simulink model "MissionServer_QDrone_Position_Control_FrSky"  (Simulink 9.1)
settings: Solver=ode2  StartTime=0.0  StopTime=inf  FixedStep=0.001  RelTol=1e-3  EnableMultiTasking=on
InitFcn:
  | set_param('MissionServer_QDrone_Position_Control_FrSky/MISSION SERVER QDRONE POSITION CONTROL/Trajectory Enable', 'sw', '0' )
  | set_param('MissionServer_QDrone_Position_Control_FrSky/MISSION SERVER QDRONE POSITION CONTROL/Command Enable', 'sw', '0' )
undefined symbols (not defined in the file): Host, qc_get_step_size
libraries: quarc_library x25, simulink x4
settings Model: Creator=Admin  LastModifiedBy=jpineros  SimulationMode=external  ExtModeTrigDuration=10000
settings SolverCC: PositivePriorityOrder=on
settings DataIOCC: SaveFormat=Dataset
settings OptimizationCC: LifeSpan=auto
settings DebuggingCC: UnderspecifiedInitializationDetection=Simplified  MergeDetectMultiDrivingBlocksExec=error
settings HardwareCC: ProdBitPerPointer=64  ProdBitPerSizeT=64  ProdBitPerPtrDiffT=64  ProdLargestAtomicFloat=Float  ProdIntDivRoundTo=Zero  ProdEndianess=LittleEndian  ProdWordSize=64  ProdHWDeviceType=Intel->x86-64 (Windows64)
settings ModelReferenceCC: PropagateSignalLabelsOutOfModel=on
settings RTWCC: SystemTargetFile=quarc_win64.tlc  TemplateMakefile=quarc_default_tmf  Description=QUARC Win64 Target  BuildConfiguration=Faster Runs
settings STFCustomTargetCC: ConcurrentExecutionCompliant=on  SystemTargetFile=quarc_win64.tlc
settings GRTTargetCC: TargetPreCompLibLocation=C:\PROGRA~3\QUARC\lib\2018a\win64\release  ParMdlRefBuildCompliant=off  CompOptLevelCompliant=off  MatFileLogging=off  CPPClassGenCompliant=off  UseToolchainInfoCompliant=off  ExtMode=on  ExtModeMexFile=quarc_comm
settings ConfigComp: CovHtmlReporting=off

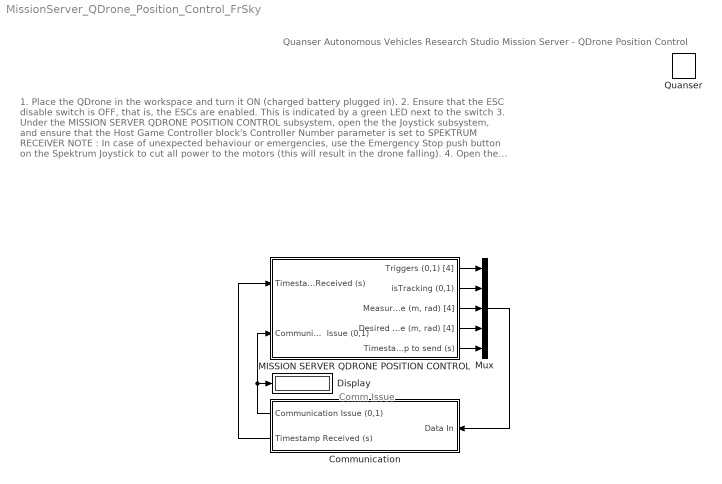
== system MissionServer_QDrone_Position_Control_FrSky ==
  note: 1. Place the QDrone in the workspace and turn it ON (charged battery plugged in).
      | 2. Ensure that the ESC disable switch is OFF, that is, the ESCs are enabled. This is indicated by a green LED next to the switch
      | 3. Under the MISSION SERVER QDRONE POSITION CONTROL subsystem, open the the Joystick subsystem, and ensure that the Host Game Controller block's Controller Number parameter is set to SPEKTRUM RECEIVER
      | NOTE : In case of unexpected behaviour or emergencies, use the Emergency Stop push button on the Spektrum Joystick to cut all power to the motors (this will result in the drone falling).
      | 4. Open the Data Server (Localization) subsystem and follow the steps there to set up the correct calibration and rigid body definition files for the selected QDrone.
      | 5. Under the QUARC menu, click on Build .
      | 6. Under the QUARC menu, click on Start . Wait for the model to start running (takes ~1 to 5 seconds for the Motive API to initialize and send localization data).
      | 7. In the MISSION SERVER QDRONE POSITION CONTROL subsystem, ensure that the isTracking? display shows 1 and that the Joystick Issue display shows 0 (joystick must be powered ON with USB dongle attached to the PC).
      | 8. Start running the Commander_Stabilizer_QDrone.mdl model.
      | 9. Arm the drone by moving the Arm/Disarm toggle to the 2 position.
      | 10. Takeoff the drone by moving the Takeoff/Land toggle to the 2 position. The QDrone should takeoff and hover.
      | 11. When finished, move the Takeoff/Land toggle to the 0 position to land the drone. The QDrone should land.
      | 12. Move the Arm/Disarm toggle to the 0 position. (The Commander_Stabilizer_QDrone.mdl model disarms the drone and stops automatically upon landing).
      | 13. Stop this model.
  note: Quanser Autonomous Vehicles Research Studio
      | Mission Server - QDrone Position Control
  note: Comm Issue
  Communication : Subsystem
  Display : Display
  MISSION SERVER QDRONE POSITION CONTROL : Subsystem
  Mux : Mux  Inputs=5
  Quanser : quarc_library/Logos/Quanser
  wires:
  Communication/2(Timestamp Received (s)) -> MISSION SERVER QDRONE POSITION CONTROL/1(Timestamp Received (s))
  MISSION SERVER QDRONE POSITION CONTROL/5(Timestamp to send (s)) -> Mux/5
  Mux/1 -> Communication/1(Data In)
  Communication/1(Communication Issue (0,1)) -> Display/1, MISSION SERVER QDRONE POSITION CONTROL/2(Communication  Issue (0,1))
  MISSION SERVER QDRONE POSITION CONTROL/3("Measured  Pose (m, rad) [4]") -> Mux/3
  MISSION SERVER QDRONE POSITION CONTROL/4("Desired  Pose (m, rad) [4]") -> Mux/4
  MISSION SERVER QDRONE POSITION CONTROL/1(Triggers (0,1) [4]) -> Mux/1
  MISSION SERVER QDRONE POSITION CONTROL/2(isTracking (0,1)) -> Mux/2

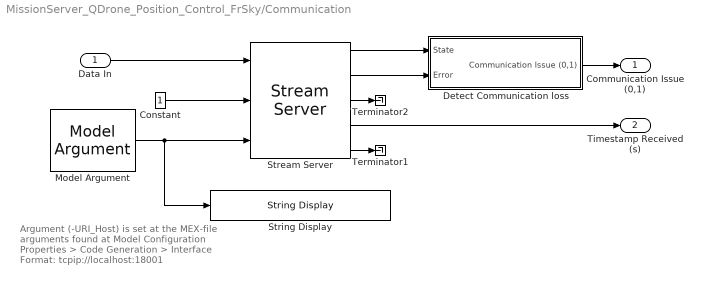
== system MissionServer_QDrone_Position_Control_FrSky/Communication ==
  note: Argument (-URI_Host) is set at the MEX-file arguments
      | found at Model Configuration Properties > Code Generation > Interface
      |
      | Format:
      | tcpip://localhost:18001
  Data In : Inport
  Constant : Constant
  Detect Communication loss : Subsystem
  Model Argument : quarc_library/Sources/Signals/Model Argument  argument_name=URI_Host  has_value=on  data_type_mode=Specify via dialog  data_type=char  max_length=80  default_value=0  variable_size=off
      settings: AttributesFormatString=(-%<argument_name>)  SourceProductName=QUARC Targets
  Stream Server : quarc_library/Communications/Basic/Stream Server  uri_source=External input port  uri=tcpip://localhost:18877  apply_uri_to_all_configs=off  send_buffer_size=1460  receive_buffer_size=1460  byte_order=little endian (Intel - LSB first)  optimization=Minimum latency  send_options=Send most recent data  receive_options=Receive most recent data  default_value=zeros(1,1)  sample_time=qc_get_step_size  active=off  implementation=Use blocking I/O in a separate thread  send_fifo_size=1000  receive_fifo_size=1000  send_priority=0  receive_priority=0  send_dimensions=off  receive_dimensions=off  max_dimensions=-1  data_type=Inherited via back propagation  type_expr=BusObject
  "String Display " : quarc_library/Strings/String Display  alignment=center  display_mode=Single line  sample_time=-1  use_new=off
      settings: SourceProductName=QUARC Targets
  Terminator1 : Terminator
  Terminator2 : Terminator
  Communication Issue (0,1) : Outport
  Timestamp Received (s) : Outport  Port=2
  wires:
  Constant/1 -> Stream Server/2
  Data In/1 -> Stream Server/1
  Stream Server/3 -> Terminator2/1
  Stream Server/5 -> Terminator1/1
  Model Argument/1 -> "String Display "/1, Stream Server/3
  Stream Server/4 -> Timestamp Received (s)/1
  Stream Server/1 -> Detect Communication loss/1(State)
  Stream Server/2 -> Detect Communication loss/2(Error)
  Detect Communication loss/1(Communication Issue (0,1)) -> Communication Issue (0,1)/1

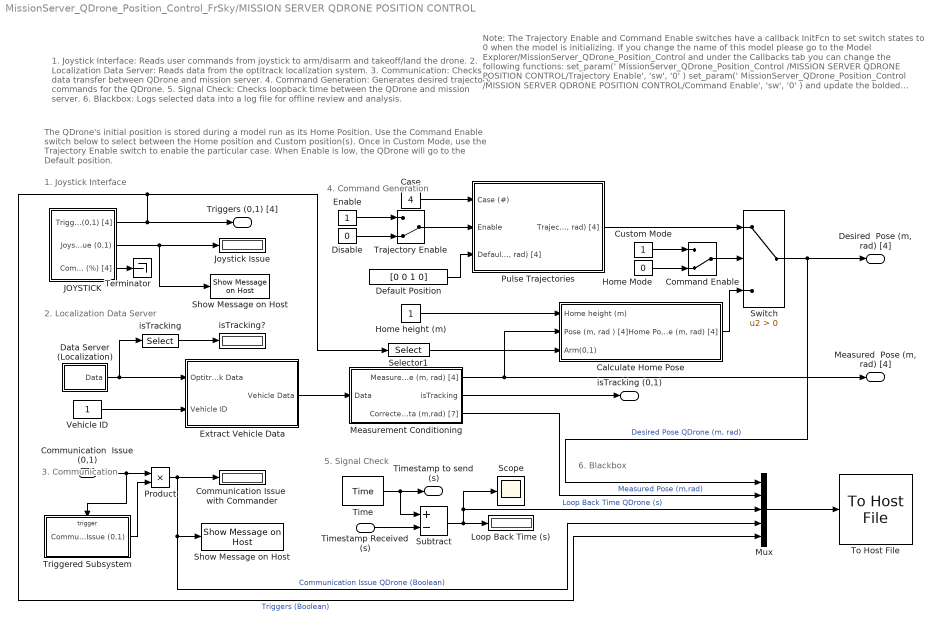
== system MissionServer_QDrone_Position_Control_FrSky/MISSION SERVER QDRONE POSITION CONTROL ==
  note: The QDrone's initial position is stored during a model run as its Home Position.
      | Use the Command Enable switch below to select between the Home position and Custom position(s).
      | Once in Custom Mode, use the Trajectory Enable switch to enable the particular case.
      | When Enable is low, the QDrone will go to the Default position.
  note: 5. Signal Check
  note: 6. Blackbox
  note: 3. Communication
  note: 2. Localization Data Server
  note: 1. Joystick Interface
  note: 4. Command Generation
  note: 1. Joystick Interface: Reads user commands from joystick to arm/disarm and takeoff/land the drone.
      | 2. Localization Data Server: Reads data from the optitrack localization system.
      | 3. Communication: Checks data transfer between QDrone and mission server.
      | 4. Command Generation: Generates desired trajectory commands for the QDrone.
      | 5. Signal Check: Checks loopback time between the QDrone and mission server.
      | 6. Blackbox: Logs selected data into a log file for offline review and analysis.
  note: Note:
      | The Trajectory Enable and Command Enable switches have a callback InitFcn to set switch states
      | to 0 when the model is initializing. If you change the name of this model please go to the Model Explorer/MissionServer_QDrone_Position_Control and under the Callbacks tab you can change the following functions:
      | set_param(' MissionServer_QDrone_Position_Control /MISSION SERVER QDRONE POSITION CONTROL/Trajectory Enable', 'sw', '0' )
      | set_param(' MissionServer_QDrone_Position_Control /MISSION SERVER QDRONE POSITION CONTROL/Command Enable', 'sw', '0' )
      | and update the bolded section with the new name of the model.
  Timestamp Received (s) : Inport
  Communication  Issue (0,1) : Inport  Port=2
  Calculate Home Pose : Subsystem
  Case : Constant  Value=4
  Command Enable : ManualSwitch  CurrentSetting=0
  Communication Issue  with Commander : Display
  Custom Mode : Constant
  "Data Server (Localization) " : Subsystem
  Default Position : Constant  Value=[0 0 1 0]
  Disable : Constant  Value=0
  Enable : Constant
  Extract Vehicle Data : Subsystem
  Home Mode : Constant  Value=0
  Home height (m) : Constant
  JOYSTICK : Subsystem
  Joystick Issue : Display
  Loop Back Time (s) : Display
  Measurement Conditioning : Subsystem
  Mux : Mux  Inputs=5
  Product : Product
  Pulse Trajectories : Subsystem
  Scope : Scope
  Selector1 : Selector  InputPortWidth=4  IndexOptions=Index vector (dialog)  Indices=[1]  OutputSizes=1
  Show Message on Host : quarc_library/Sinks/Error Handling/Show Message on Host  message_type=Fixed error message  message_icon=Warning  message=Mission Server: Communication Issue with QDrone
      settings: AttributesFormatString="\"%<message>\""  SourceProductName=QUARC Targets
  "Show Message on Host " : quarc_library/Sinks/Error Handling/Show Message on Host  message_type=Fixed error message  message_icon=Warning  message=Mission Server: Joystick Disconnected
      settings: AttributesFormatString="\"%<message>\""  SourceProductName=QUARC Targets
  Subtract : Sum  Inputs=+-
  Switch : Switch  Criteria=u2 > Threshold
  Terminator : Terminator
  Time : quarc_library/Sources/Time/Time  time_source=Wall clock  sample_time=qc_get_step_size
  To Host File : quarc_library/Sinks/To Host/To Host File  file_name=saved_data/%m/Mission_Server_%{date}_%{time}.mat  variable_name=mission_server_data  decimation=1  sample_time=-1  file_format=MAT-file v.5  options=No header or footer  append=off  final_file_name=saved_data/MissionServer_QDrone_Position_Control_FrSky/Mission_Server_20-Jan-2022_08-53-09.mat  bitrate=2000000
  Trajectory Enable : ManualSwitch  CurrentSetting=0
  Triggered Subsystem : Subsystem  TreatAsAtomicUnit=on
  Vehicle ID : Constant
  isTracking : Selector  InputPortWidth=7  IndexOptions=Index vector (dialog)  Indices=[7]  OutputSizes=1
  isTracking? : Display
  Triggers (0,1) [4] : Outport
  isTracking (0,1) : Outport  Port=2
  "Measured  Pose (m, rad) [4]" : Outport  Port=3
  "Desired  Pose (m, rad) [4]" : Outport  Port=4
  Timestamp to send (s) : Outport  Port=5
  wires:
  Communication  Issue (0,1)/1 -> Product/1, Triggered Subsystem/Trigger
  isTracking/1 -> isTracking?/1
  JOYSTICK/2(Joystick Issue (0,1)) -> "Show Message on Host "/1, Joystick Issue/1
  JOYSTICK/3(Commands (%) [4]) -> Terminator/1
  JOYSTICK/1(Triggers (0,1) [4]) -> Mux/5, Selector1/1, Triggers (0,1) [4]/1  "Triggers (Boolean)"
  Time/1 -> Subtract/1, Timestamp to send (s)/1
  Timestamp Received (s)/1 -> Subtract/2
  Subtract/1 -> Mux/3, Scope/1, Loop Back Time (s)/1  "Loop Back Time QDrone (s)"
  Switch/1 -> Mux/1, "Desired  Pose (m, rad) [4]"/1  "Desired Pose QDrone (m, rad)"
  Measurement Conditioning/2(isTracking) -> isTracking (0,1)/1
  Measurement Conditioning/1("Measured Pose (m, rad) [4]") -> Calculate Home Pose/2("Pose (m, rad ) [4]"), "Measured  Pose (m, rad) [4]"/1
  "Data Server (Localization) "/1(Data) -> Extract Vehicle Data/1(Optitrack Data), isTracking/1
  Vehicle ID/1 -> Extract Vehicle Data/2(Vehicle ID)
  Extract Vehicle Data/1(Vehicle Data) -> Measurement Conditioning/1(Data)
  Calculate Home Pose/1("Home Pose (m, rad) [4]") -> Switch/3
  Home height (m)/1 -> Calculate Home Pose/1(Home height (m))
  Triggered Subsystem/1(Communication Issue (0,1)) -> Product/2
  Product/1 -> Communication Issue  with Commander/1, Mux/4, Show Message on Host/1  "Communication Issue QDrone (Boolean)"
  Mux/1 -> To Host File/1
  Custom Mode/1 -> Command Enable/1
  Command Enable/1 -> Switch/2
  Home Mode/1 -> Command Enable/2
  Enable/1 -> Trajectory Enable/1
  Disable/1 -> Trajectory Enable/2
  Trajectory Enable/1 -> Pulse Trajectories/2(Enable)
  Default Position/1 -> Pulse Trajectories/3("Default (m, rad) [4]")
  Case/1 -> Pulse Trajectories/1(Case (#))
  Pulse Trajectories/1("Trajectory (m, rad) [4]") -> Switch/1
  Selector1/1 -> Calculate Home Pose/3(Arm(0,1))
  Measurement Conditioning/3(Corrected Pose Data (m,rad) [7]) -> Mux/2  "Measured Pose (m,rad)"

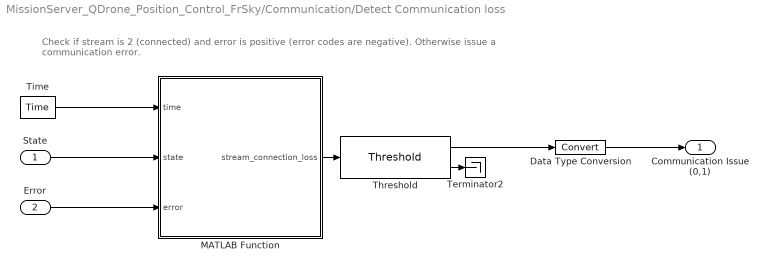
== system MissionServer_QDrone_Position_Control_FrSky/Communication/Detect Communication loss ==
  note: Check if stream is 2 (connected) and error is positive (error codes are negative). Otherwise issue a communication error.
  State : Inport
  Error : Inport  Port=2
  Data Type Conversion : DataTypeConversion
  MATLAB Function : MATLAB Function  TreatAsAtomicUnit=on
  Terminator2 : Terminator
  Threshold : quarc_library/Discontinuities/Threshold  operator=>=  param_src=Specify via dialog  threshold=0.5  duration=0.1
      settings: SourceProductName=QUARC Targets
  Time : quarc_library/Sources/Time/Time  time_source=Wall clock  sample_time=qc_get_step_size
  Communication Issue (0,1) : Outport
  wires:
  Error/1 -> MATLAB Function/3(error)
  MATLAB Function/1(stream_connection_loss) -> Threshold/1
  State/1 -> MATLAB Function/2(state)
  Time/1 -> MATLAB Function/1(time)
  Threshold/2 -> Terminator2/1
  Data Type Conversion/1 -> Communication Issue (0,1)/1
  Threshold/1 -> Data Type Conversion/1

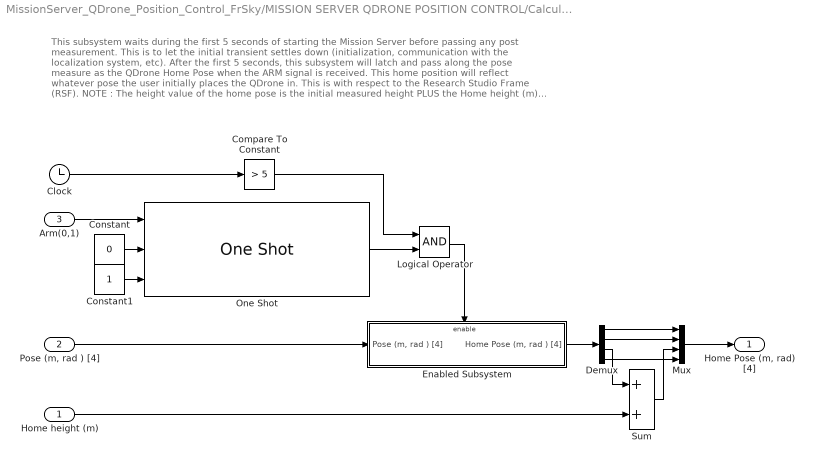
== system MissionServer_QDrone_Position_Control_FrSky/MISSION SERVER QDRONE POSITION CONTROL/Calculate Home Pose ==
  note: This subsystem waits during the first 5 seconds of starting the Mission Server before passing any post measurement.
      | This is to let the initial transient settles down (initialization, communication with the localization system, etc).
      | After the first 5 seconds, this subsystem will latch and pass along the pose measure as the QDrone Home Pose when
      | the ARM signal is received.
      | This home position will reflect whatever pose the user initially places the QDrone in.
      | This is with respect to the Research Studio Frame (RSF).
      |
      | NOTE : The height value of the home pose is the initial measured height PLUS the Home height (m) input value.
  Home height (m) : Inport
  "Pose (m, rad ) [4]" : Inport  Port=2
  Arm(0,1) : Inport  Port=3
  Clock : Clock
  Compare To Constant : simulink/Logic and Bit Operations/Compare To Constant  relop=>  const=5  OutDataTypeStr=boolean
  Constant : Constant  Value=0
  Constant1 : Constant
  Demux : Demux
  Enabled Subsystem : Subsystem  TreatAsAtomicUnit=on
  Logical Operator : Logic  AllPortsSameDT=off  OutDataTypeStr=boolean
  Mux : Mux
  One Shot : quarc_library/Discontinuities/One Shot  trigger_type=Rising edge  redun_pulse=Ignore extraneous pulse  width_source=Specify via dialog  pulse_width=1/qc_get_step_size
      settings: SourceProductName=QUARC Targets
  Sum : Sum
  "Home Pose (m, rad) [4]" : Outport
  wires:
  Constant/1 -> One Shot/2
  Constant1/1 -> One Shot/3
  Arm(0,1)/1 -> One Shot/1
  One Shot/1 -> Logical Operator/2
  "Pose (m, rad ) [4]"/1 -> Enabled Subsystem/1("Pose (m, rad ) [4] ")
  Clock/1 -> Compare To Constant/1
  Compare To Constant/1 -> Logical Operator/1
  Logical Operator/1 -> Enabled Subsystem/Enable
  Enabled Subsystem/1("Home Pose (m, rad ) [4]") -> Demux/1
  Demux/1 -> Mux/1
  Demux/2 -> Mux/2
  Demux/4 -> Mux/4
  Demux/3 -> Sum/1
  Sum/1 -> Mux/3
  Home height (m)/1 -> Sum/2
  Mux/1 -> "Home Pose (m, rad) [4]"/1

== system MissionServer_QDrone_Position_Control_FrSky/MISSION SERVER QDRONE POSITION CONTROL/Data Server (Localization)  ==
  note: Double-click on the OptiTrack Trackables block.
      |
      | Click on the ... icon under Calibration file: and select the .cal file
      | created when calibrating the Optitrack cameras
      |
      | Click on the ... icon under Trackables definition file: and select
      | the trackables file created when defining rigid bodies (for the
      | QDrone you are about to use)
  Convention Correction (Motive Frame to Research Studio Frame) : Subsystem
  Data Type Conversion : DataTypeConversion
  Mux : Mux  Inputs=3
  OptiTrack Trackables : quarc_library/Devices/Third-Party/NaturalPoint/OptiTrack/OptiTrack Trackables  calibration_file=C:\Users\user\Documents\optitrack\03-06-2020\CalibrationResult 2020-03-06 9.cal  rigid_body_file=C:\Users\user\Documents\optitrack\02-27-2020\Motive Profile - 2020-03-06.motive  rigid_body_ids=[1]  sample_time=qc_get_step_size*10  active=off
      settings: SourceProductName=QUARC Targets
  Rate Transition2 : RateTransition
  Terminator : Terminator
  Data : Outport
  wires:
  Mux/1 -> Rate Transition2/1
  Convention Correction (Motive Frame to Research Studio Frame)/1(xyz_RSF (m) [3]) -> Mux/1
  Convention Correction (Motive Frame to Research Studio Frame)/2(rot_RSF (rad) [3]) -> Mux/2
  Data Type Conversion/1 -> Mux/3
  OptiTrack Trackables/1 -> Convention Correction (Motive Frame to Research Studio Frame)/1(xyz_MF (m) [3])
  OptiTrack Trackables/2 -> Terminator/1
  OptiTrack Trackables/3 -> Convention Correction (Motive Frame to Research Studio Frame)/2(rot_MF (rad) [3])
  OptiTrack Trackables/4 -> Data Type Conversion/1
  Rate Transition2/1 -> Data/1

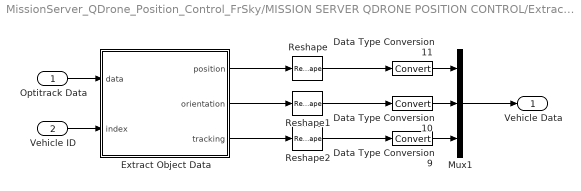
== system MissionServer_QDrone_Position_Control_FrSky/MISSION SERVER QDRONE POSITION CONTROL/Extract Vehicle Data ==
  Optitrack Data : Inport
  Vehicle ID : Inport  Port=2
  Data Type Conversion10 : DataTypeConversion
  Data Type Conversion11 : DataTypeConversion
  Data Type Conversion9 : DataTypeConversion
  Extract Object Data : MATLAB Function  TreatAsAtomicUnit=on
  Mux1 : Mux  Inputs=3
  Reshape : Reshape
  Reshape1 : Reshape
  Reshape2 : Reshape
  Vehicle Data : Outport
  wires:
  Vehicle ID/1 -> Extract Object Data/2(index)
  Optitrack Data/1 -> Extract Object Data/1(data)
  Mux1/1 -> Vehicle Data/1
  Extract Object Data/1(position) -> Reshape/1
  Extract Object Data/3(tracking) -> Reshape2/1
  Extract Object Data/2(orientation) -> Reshape1/1
  Data Type Conversion11/1 -> Mux1/1
  Data Type Conversion10/1 -> Mux1/2
  Data Type Conversion9/1 -> Mux1/3
  Reshape/1 -> Data Type Conversion11/1
  Reshape1/1 -> Data Type Conversion10/1
  Reshape2/1 -> Data Type Conversion9/1

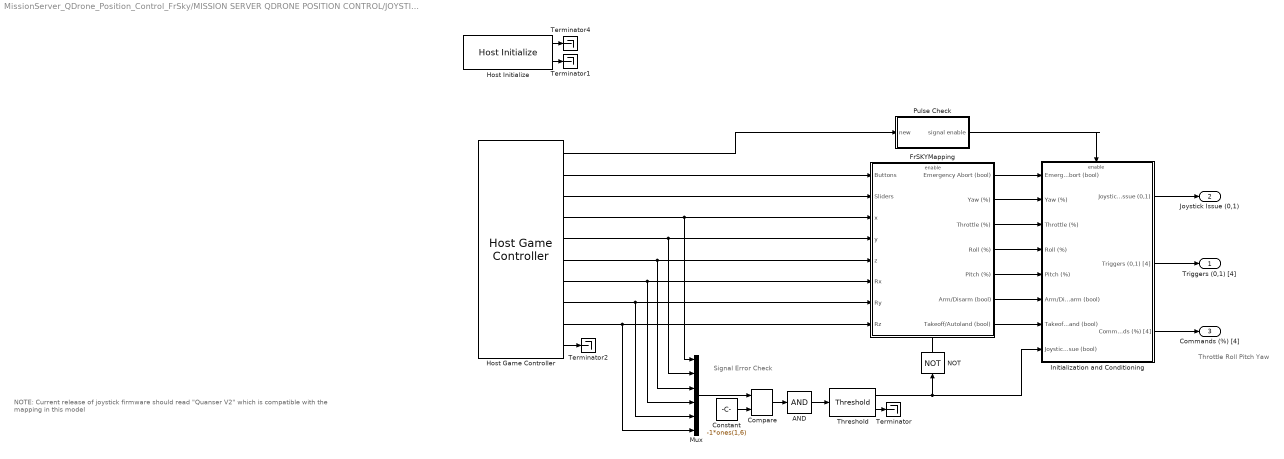
== system MissionServer_QDrone_Position_Control_FrSky/MISSION SERVER QDRONE POSITION CONTROL/JOYSTICK ==
  note: Signal Error Check
  note: Throttle
      | Roll
      | Pitch
      | Yaw
  note: NOTE: Current release of joystick firmware should read "Quanser V2" which is compatible with the mapping in this model
  AND : Logic  Inputs=1  AllPortsSameDT=off  OutDataTypeStr=boolean
  Compare : quarc_library/Logic Operations/Compare  operator===  output_data_type=boolean
      settings: SourceProductName=QUARC Targets
  Constant : Constant  Value=-1*ones(1,6)
  FrSKYMapping : Subsystem
  Host Game Controller : quarc_library/Devices/Peripherals/Host/Host Game Controller  object_name=Host-1  controller=1  buffer_size=20  deadzone=[]  saturation=[]  sample_time=qc_get_step_size  auto_center=off  enabled=on  debug_mode=off
      settings: SourceProductName=QUARC Targets
  Host Initialize : quarc_library/Devices/Peripherals/Host/Host Initialize  object_name=Host-1  uri_source=Use external mode communications  uri=tcpip://localhost:18001  apply_uri_to_all_configs=on  send_buffer_size=1000  receive_buffer_size=1000  thread_priority=0  run_client=on  use_window=off  window_position=[]  sample_time=qc_get_step_size  active=on
      settings: SourceProductName=QUARC Targets
  Initialization and Conditioning : Subsystem  TreatAsAtomicUnit=on
  Mux : Mux  Inputs=6
  NOT : Logic  Operator=NOT  IconShape=distinctive  AllPortsSameDT=off  OutDataTypeStr=boolean
  Pulse Check : Subsystem  TreatAsAtomicUnit=on
  Terminator{,1..2,4} (4 alike) : Terminator
  Threshold : quarc_library/Discontinuities/Threshold  operator=>=  param_src=Specify via dialog  threshold=0.5  duration=0.2
      settings: SourceProductName=QUARC Targets
  Triggers (0,1) [4] : Outport
  Joystick Issue (0,1) : Outport  Port=2
  Commands (%) [4] : Outport  Port=3
  wires:
  FrSKYMapping/2(Yaw (%)) -> Initialization and Conditioning/2(Yaw (%))
  FrSKYMapping/3(Throttle (%)) -> Initialization and Conditioning/3(Throttle (%))
  FrSKYMapping/1(Emergency Abort (bool)) -> Initialization and Conditioning/1(Emergency Abort (bool))
  FrSKYMapping/5(Pitch (%)) -> Initialization and Conditioning/5(Pitch (%))
  FrSKYMapping/6("Arm/Disarm (bool) ") -> Initialization and Conditioning/6(Arm/Disarm (bool))
  FrSKYMapping/4(Roll (%)) -> Initialization and Conditioning/4(Roll (%))
  Host Game Controller/1 -> Pulse Check/1(new)
  Pulse Check/1(signal enable) -> Initialization and Conditioning/Enable
  FrSKYMapping/7(Takeoff/Autoland (bool)) -> Initialization and Conditioning/7(Takeoff/AutoLand (bool))
  Host Game Controller/4 -> Mux/1, FrSKYMapping/3(x)
  Host Game Controller/5 -> Mux/2, FrSKYMapping/4(y)
  Host Game Controller/6 -> Mux/3, FrSKYMapping/5(z)
  Host Game Controller/7 -> Mux/4, FrSKYMapping/6(Rx)
  Host Game Controller/8 -> Mux/5, FrSKYMapping/7(Ry)
  Host Game Controller/9 -> Mux/6, FrSKYMapping/8(Rz)
  Mux/1 -> Compare/1
  Constant/1 -> Compare/2
  Compare/1 -> AND/1
  Threshold/2 -> Terminator/1
  Host Game Controller/2 -> FrSKYMapping/1(Buttons)
  Host Game Controller/3 -> FrSKYMapping/2(Sliders)
  Threshold/1 -> NOT/1, Initialization and Conditioning/8(Joystick Issue (bool))
  NOT/1 -> FrSKYMapping/Enable
  AND/1 -> Threshold/1
  Initialization and Conditioning/3(Commands (%) [4]) -> Commands (%) [4]/1
  Initialization and Conditioning/2(Triggers (0,1) [4]) -> Triggers (0,1) [4]/1
  Host Initialize/2 -> Terminator1/1
  Host Initialize/1 -> Terminator4/1
  Host Game Controller/10 -> Terminator2/1
  Initialization and Conditioning/1(Joystick Issue (0,1)) -> Joystick Issue (0,1)/1

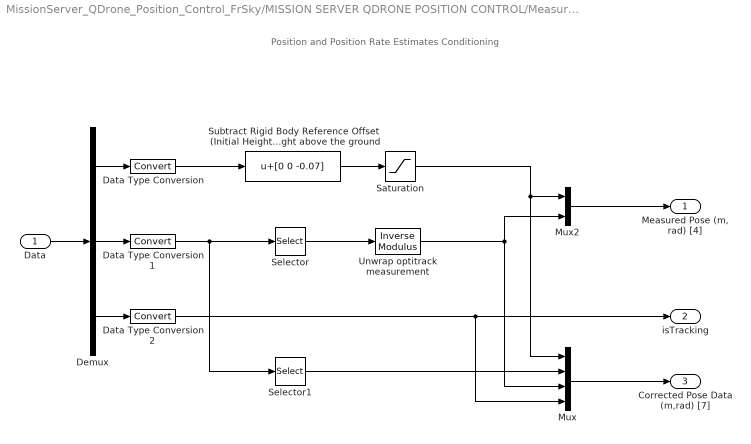
== system MissionServer_QDrone_Position_Control_FrSky/MISSION SERVER QDRONE POSITION CONTROL/Measurement Conditioning ==
  note: Position and Position Rate Estimates Conditioning
  Data : Inport
  Data Type Conversion : DataTypeConversion
  Data Type Conversion1 : DataTypeConversion
  Data Type Conversion2 : DataTypeConversion
  Demux : Demux  Outputs=[3 3 1]
  Mux : Mux
  Mux2 : Mux  Inputs=[3 1]
  Saturation : Saturate  UpperLimit=[2 2 5]  LowerLimit=[-2 -2 0]
  Selector : Selector  InputPortWidth=3  IndexOptions=Index vector (dialog)  Indices=[3]  OutputSizes=1
  Selector1 : Selector  InputPortWidth=3  IndexOptions=Index vector (dialog)  Indices=[1 2]  OutputSizes=1
  Subtract Rigid Body Reference Offset  (Initial Height)  to get height above the ground : Bias  Bias=[0 0 -0.07]
  Unwrap optitrack measurement : quarc_library/Discontinuities/Inverse Modulus  modulus=2*pi  output_derivative=off  output_revolutions=off  max_x=Inf  min_x=-Inf
  "Measured Pose (m, rad) [4]" : Outport
  isTracking : Outport  Port=2
  Corrected Pose Data (m,rad) [7] : Outport  Port=3
  wires:
  Demux/2 -> Data Type Conversion1/1
  Demux/1 -> Data Type Conversion/1
  Demux/3 -> Data Type Conversion2/1
  Mux2/1 -> "Measured Pose (m, rad) [4]"/1
  Data/1 -> Demux/1
  Data Type Conversion2/1 -> Mux/4, isTracking/1
  Subtract Rigid Body Reference Offset  (Initial Height)  to get height above the ground/1 -> Saturation/1
  Saturation/1 -> Mux2/1, Mux/1
  Data Type Conversion1/1 -> Selector1/1, Selector/1
  Selector/1 -> Unwrap optitrack measurement/1
  Data Type Conversion/1 -> Subtract Rigid Body Reference Offset  (Initial Height)  to get height above the ground/1
  Unwrap optitrack measurement/1 -> Mux/3, Mux2/2
  Mux/1 -> Corrected Pose Data (m,rad) [7]/1
  Selector1/1 -> Mux/2

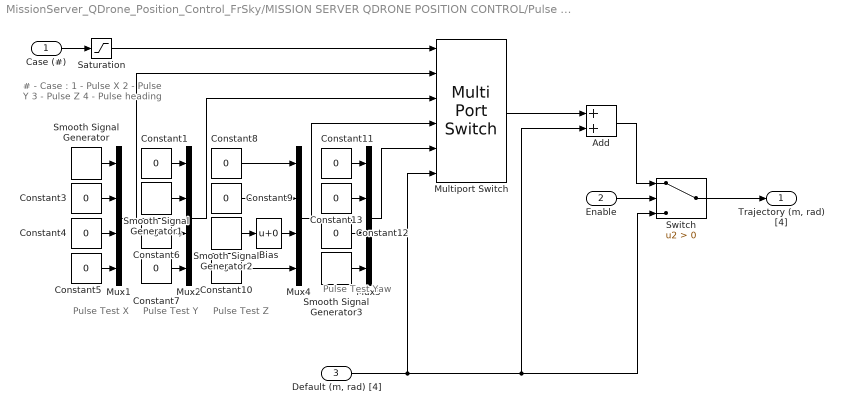
== system MissionServer_QDrone_Position_Control_FrSky/MISSION SERVER QDRONE POSITION CONTROL/Pulse Trajectories ==
  note: Pulse
      | Test Y
  note: Pulse
      | Test X
  note: Pulse
      | Test Z
  note: Pulse
      | Test
      | Yaw
  note: # - Case :
      | 1 - Pulse X
      | 2 - Pulse Y
      | 3 - Pulse Z
      | 4 - Pulse heading
  Case (#) : Inport
  Enable : Inport  Port=2
  "Default (m, rad) [4]" : Inport  Port=3
  Add : Sum
  Bias : Bias
  Constant{1,3..13} (12 alike) : Constant  Value=0
  Multiport Switch : MultiPortSwitch  Inputs=5
  Mux{1..2,4..5} (4 alike) : Mux  Inputs=[1 1 1 1]
  Saturation : Saturate  UpperLimit=5  LowerLimit=1
  Smooth Signal Generator : quarc_library/Sources/Signals/Smooth Signal Generator  signal_type=Square  source=Internal (dialog parameters)  amplitude=0.75  frequency=0.05  initial_phase=0  sample_time=qc_get_step_size  output_cos=off
      settings: SourceProductName=QUARC Targets
  Smooth Signal Generator1 : quarc_library/Sources/Signals/Smooth Signal Generator  signal_type=Square  source=Internal (dialog parameters)  amplitude=0.75  frequency=0.05  initial_phase=0  sample_time=qc_get_step_size  output_cos=off
      settings: SourceProductName=QUARC Targets
  Smooth Signal Generator2 : quarc_library/Sources/Signals/Smooth Signal Generator  signal_type=Square  source=Internal (dialog parameters)  amplitude=0.5  frequency=0.05  initial_phase=0  sample_time=qc_get_step_size  output_cos=off
      settings: SourceProductName=QUARC Targets
  Smooth Signal Generator3 : quarc_library/Sources/Signals/Smooth Signal Generator  signal_type=Square  source=Internal (dialog parameters)  amplitude=pi/4  frequency=0.05  initial_phase=0  sample_time=qc_get_step_size  output_cos=off
      settings: SourceProductName=QUARC Targets
  Switch : Switch  Criteria=u2 > Threshold
  "Trajectory (m, rad) [4]" : Outport
  wires:
  Constant3/1 -> Mux1/2
  Smooth Signal Generator/1 -> Mux1/1
  Constant5/1 -> Mux1/4
  Constant4/1 -> Mux1/3
  Mux1/1 -> Multiport Switch/2
  Case (#)/1 -> Saturation/1
  Mux2/1 -> Multiport Switch/3
  Constant6/1 -> Mux2/3
  Constant7/1 -> Mux2/4
  Constant1/1 -> Mux2/1
  Smooth Signal Generator1/1 -> Mux2/2
  Constant9/1 -> Mux4/2
  Constant8/1 -> Mux4/1
  Constant10/1 -> Mux4/4
  Smooth Signal Generator2/1 -> Bias/1
  Bias/1 -> Mux4/3
  Constant13/1 -> Mux5/2
  Constant11/1 -> Mux5/1
  Smooth Signal Generator3/1 -> Mux5/4
  Constant12/1 -> Mux5/3
  Mux4/1 -> Multiport Switch/4
  Mux5/1 -> Multiport Switch/5
  Saturation/1 -> Multiport Switch/1
  "Default (m, rad) [4]"/1 -> Add/2, Switch/3, Multiport Switch/6
  Switch/1 -> "Trajectory (m, rad) [4]"/1
  Enable/1 -> Switch/2
  Multiport Switch/1 -> Add/1
  Add/1 -> Switch/1

== system MissionServer_QDrone_Position_Control_FrSky/MISSION SERVER QDRONE POSITION CONTROL/Triggered Subsystem ==
  note: This looks for the first falling edge of the communication issue before allowing a communication issue to be triggered,
      | because the mission server model starts first.
  Trigger : TriggerPort  TriggerType=falling  VariantControl=Variant
  Add : Sum
  Compare To Constant : simulink/Logic and Bit Operations/Compare To Constant  relop=>=  const=1  OutDataTypeStr=boolean
  Constant : Constant
  Memory : Memory  InheritSampleTime=on
  Communication Issue (0,1) : Outport  InitialOutput=0
  wires:
  Constant/1 -> Add/1
  Memory/1 -> Add/2
  Add/1 -> Compare To Constant/1, Memory/1
  Compare To Constant/1 -> Communication Issue (0,1)/1

== system MissionServer_QDrone_Position_Control_FrSky/MISSION SERVER QDRONE POSITION CONTROL/Calculate Home Pose/Enabled Subsystem ==
  "Pose (m, rad ) [4] " : Inport
  Enable : EnablePort
  "Home Pose (m, rad ) [4]" : Outport
  wires:
  "Pose (m, rad ) [4] "/1 -> "Home Pose (m, rad ) [4]"/1

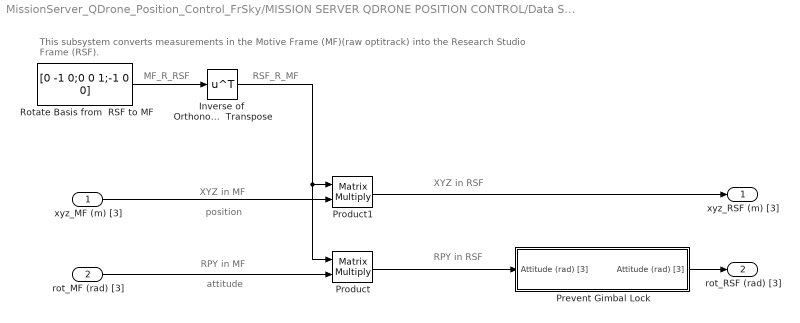
== system MissionServer_QDrone_Position_Control_FrSky/MISSION SERVER QDRONE POSITION CONTROL/Data Server (Localization) /Convention Correction (Motive Frame to Research Studio Frame) ==
  note: MF_R_RSF
  note: This subsystem converts measurements in the Motive Frame (MF)(raw optitrack) into the Research Studio Frame (RSF).
  note: RSF_R_MF
  note: XYZ in MF
  note: RPY in MF
  note: position
  note: attitude
  note: XYZ in RSF
  note: RPY in RSF
  xyz_MF (m) [3] : Inport
  rot_MF (rad) [3] : Inport  Port=2
  Inverse of  Orthonormal  Matrix is its  Transpose : Math  Operator=transpose  SaturateOnIntegerOverflow=on
  Prevent Gimbal Lock : Subsystem
  Product : Product  Multiplication=Matrix(*)
  Product1 : Product  Multiplication=Matrix(*)
  Rotate Basis from  RSF to MF : Constant  Value=[0 -1 0;0 0 1;-1 0 0]
  xyz_RSF (m) [3] : Outport
  rot_RSF (rad) [3] : Outport  Port=2
  wires:
  Rotate Basis from  RSF to MF/1 -> Inverse of  Orthonormal  Matrix is its  Transpose/1
  xyz_MF (m) [3]/1 -> Product1/2
  Inverse of  Orthonormal  Matrix is its  Transpose/1 -> Product1/1, Product/1
  rot_MF (rad) [3]/1 -> Product/2
  Product1/1 -> xyz_RSF (m) [3]/1
  Product/1 -> Prevent Gimbal Lock/1(Attitude (rad) [3])
  Prevent Gimbal Lock/1("Attitude (rad) [3] ") -> rot_RSF (rad) [3]/1

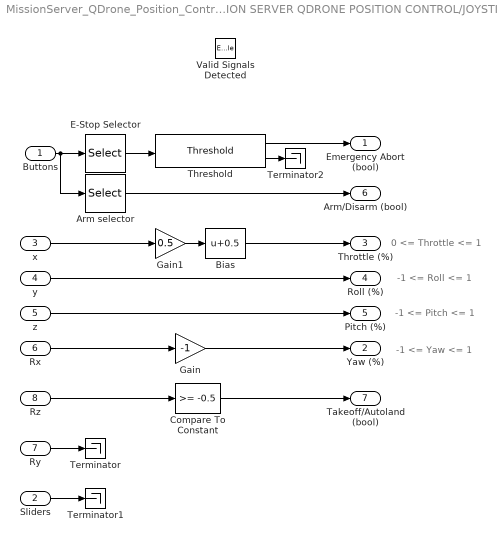
== system MissionServer_QDrone_Position_Control_FrSky/MISSION SERVER QDRONE POSITION CONTROL/JOYSTICK/FrSKYMapping ==
  note: -1 <= Yaw <= 1
  note: 0 <= Throttle <= 1
  note: -1 <= Roll <= 1
  note: -1 <= Pitch <= 1
  Buttons : Inport
  Sliders : Inport  Port=2
  x : Inport  Port=3
  y : Inport  Port=4
  z : Inport  Port=5
  Rx : Inport  Port=6
  Ry : Inport  Port=7
  Rz : Inport  Port=8
  Valid Signals Detected : EnablePort
  Arm selector : Selector  InputPortWidth=32  IndexOptions=Index vector (dialog)  Indices=[2]  OutputSizes=1
  Bias : Bias  Bias=0.5
  Compare To Constant : simulink/Logic and Bit Operations/Compare To Constant  relop=>=  const=-0.5  OutDataTypeStr=boolean
  E-Stop Selector : Selector  InputPortWidth=32  IndexOptions=Index vector (dialog)  Indices=[1]  OutputSizes=1
  Gain : Gain  Gain=-1
  Gain1 : Gain  Gain=0.5
  Terminator : Terminator
  Terminator1 : Terminator
  Terminator2 : Terminator
  Threshold : quarc_library/Discontinuities/Threshold  operator=>=  param_src=Specify via dialog  threshold=0.5  duration=0.2
      settings: SourceProductName=QUARC Targets
  Emergency Abort (bool) : Outport
  Yaw (%) : Outport  Port=2
  Throttle (%) : Outport  Port=3
  Roll (%) : Outport  Port=4
  Pitch (%) : Outport  Port=5
  "Arm/Disarm (bool) " : Outport  Port=6
  Takeoff/Autoland (bool) : Outport  Port=7
  wires:
  Buttons/1 -> Arm selector/1, E-Stop Selector/1
  Arm selector/1 -> "Arm/Disarm (bool) "/1
  x/1 -> Gain1/1
  y/1 -> Roll (%)/1
  z/1 -> Pitch (%)/1
  Rx/1 -> Gain/1
  Ry/1 -> Terminator/1
  Sliders/1 -> Terminator1/1
  E-Stop Selector/1 -> Threshold/1
  Rz/1 -> Compare To Constant/1
  Compare To Constant/1 -> Takeoff/Autoland (bool)/1
  Threshold/1 -> Emergency Abort (bool)/1
  Threshold/2 -> Terminator2/1
  Gain/1 -> Yaw (%)/1
  Gain1/1 -> Bias/1
  Bias/1 -> Throttle (%)/1

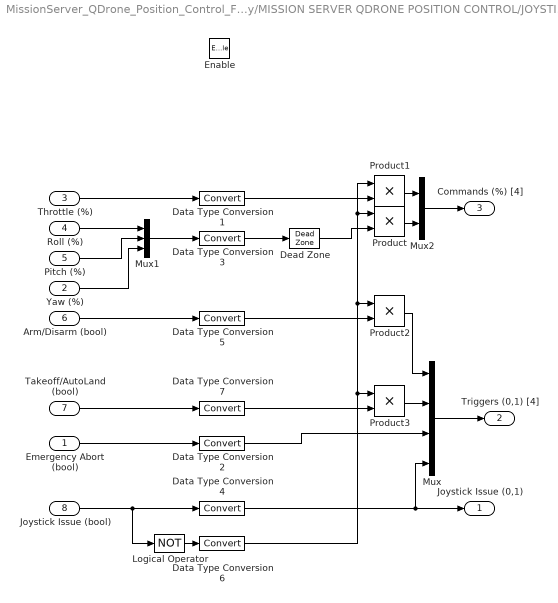
== system MissionServer_QDrone_Position_Control_FrSky/MISSION SERVER QDRONE POSITION CONTROL/JOYSTICK/Initialization and Conditioning ==
  Emergency Abort (bool) : Inport
  Yaw (%) : Inport  Port=2
  Throttle (%) : Inport  Port=3
  Roll (%) : Inport  Port=4
  Pitch (%) : Inport  Port=5
  Arm/Disarm (bool) : Inport  Port=6
  Takeoff/AutoLand (bool) : Inport  Port=7
  Joystick Issue (bool) : Inport  Port=8
  Enable : EnablePort  StatesWhenEnabling=reset
  Data Type Conversion{1..7} (7 alike) : DataTypeConversion
  Dead Zone : DeadZone  LowerValue=-0.01  UpperValue=0.01  SaturateOnIntegerOverflow=on
  Logical Operator : Logic  Operator=NOT  AllPortsSameDT=off  OutDataTypeStr=boolean
  Mux : Mux
  Mux1 : Mux  Inputs=3
  Mux2 : Mux  Inputs=2
  Product{,1..3} (4 alike) : Product
  Joystick Issue (0,1) : Outport  InitialOutput=0
  Triggers (0,1) [4] : Outport  Port=2  InitialOutput=0
  Commands (%) [4] : Outport  Port=3  InitialOutput=0
  wires:
  Joystick Issue (bool)/1 -> Data Type Conversion4/1, Logical Operator/1
  Mux1/1 -> Data Type Conversion3/1
  Throttle (%)/1 -> Data Type Conversion1/1
  Roll (%)/1 -> Mux1/1
  Pitch (%)/1 -> Mux1/2
  Yaw (%)/1 -> Mux1/3
  Data Type Conversion4/1 -> Mux/4, Joystick Issue (0,1)/1
  Emergency Abort (bool)/1 -> Data Type Conversion2/1
  Data Type Conversion3/1 -> Dead Zone/1
  Arm/Disarm (bool)/1 -> Data Type Conversion5/1
  Mux/1 -> Triggers (0,1) [4]/1
  Data Type Conversion2/1 -> Mux/3
  Logical Operator/1 -> Data Type Conversion6/1
  Product/1 -> Mux2/2
  Product1/1 -> Mux2/1
  Data Type Conversion1/1 -> Product1/2
  Dead Zone/1 -> Product/2
  Data Type Conversion6/1 -> Product1/1, Product/1, Product2/1, Product3/1
  Product2/1 -> Mux/1
  Data Type Conversion5/1 -> Product2/2
  Takeoff/AutoLand (bool)/1 -> Data Type Conversion7/1
  Product3/1 -> Mux/2
  Data Type Conversion7/1 -> Product3/2
  Mux2/1 -> Commands (%) [4]/1

== system MissionServer_QDrone_Position_Control_FrSky/MISSION SERVER QDRONE POSITION CONTROL/JOYSTICK/Pulse Check ==
  note: For this subsystem we will count the number of new pulses. The data can be considered enabled once the count of new signals has gone beyond 1. This will enable the Initializing and conditioning subsystem.
  new : Inport
  Compare : quarc_library/Logic Operations/Compare  operator=>=  output_data_type=boolean
      settings: SourceProductName=QUARC Targets
  Pulse Check : Constant
  "pulse count " : Subsystem  TreatAsAtomicUnit=on
  signal enable : Outport  InitialOutput=0
  wires:
  Compare/1 -> signal enable/1
  Pulse Check/1 -> Compare/2
  new/1 -> "pulse count "/Trigger
  "pulse count "/1(Number of Pulses) -> Compare/1

== system MissionServer_QDrone_Position_Control_FrSky/MISSION SERVER QDRONE POSITION CONTROL/Data Server (Localization) /Convention Correction (Motive Frame to Research Studio Frame)/Prevent Gimbal Lock ==
  note: Remapping the rotation order to prevent gimbal lock
      | in heading/yaw due to Euler singularity condition
  Attitude (rad) [3] : Inport
  Demux : Demux  Outputs=3
  Euler Angles from Rotation Matrix (Relative ZYX) : quarc_library/Math Operations/Matrices/Euler Angles from Rotation Matrix  menu_order=Relative Z-Y-X
      settings: SourceProductName=QUARC Targets
  Euler Angles to Rotation Matrix (Relative YZX) : quarc_library/Math Operations/Matrices/Euler Angles to Rotation Matrix  menu_order=Relative Y-Z-X
      settings: SourceProductName=QUARC Targets
  Mux : Mux  Inputs=3
  "Attitude (rad) [3] " : Outport
  wires:
  Euler Angles from Rotation Matrix (Relative ZYX)/2 -> Mux/2
  Euler Angles from Rotation Matrix (Relative ZYX)/1 -> Mux/3
  Euler Angles from Rotation Matrix (Relative ZYX)/3 -> Mux/1
  Euler Angles to Rotation Matrix (Relative YZX)/1 -> Euler Angles from Rotation Matrix (Relative ZYX)/1
  Attitude (rad) [3]/1 -> Demux/1
  Mux/1 -> "Attitude (rad) [3] "/1
  Demux/2 -> Euler Angles to Rotation Matrix (Relative YZX)/1
  Demux/3 -> Euler Angles to Rotation Matrix (Relative YZX)/2
  Demux/1 -> Euler Angles to Rotation Matrix (Relative YZX)/3

== system MissionServer_QDrone_Position_Control_FrSky/MISSION SERVER QDRONE POSITION CONTROL/JOYSTICK/Pulse Check/pulse count  ==
  Trigger : TriggerPort  TriggerType=either  VariantControl=Variant
  Constant1 : Constant  Value=0
  Increment Stored Integer : simulink/Additional Math & Discrete/Additional Math: Increment - Decrement/Increment Stored Integer
  Sum : Sum  Inputs=|++
  Unit Delay : UnitDelay  SampleTime=-1
  Number of Pulses : Outport
  wires:
  Constant1/1 -> Sum/1
  Sum/1 -> Increment Stored Integer/1
  Unit Delay/1 -> Sum/2
  Increment Stored Integer/1 -> Unit Delay/1, Number of Pulses/1

== matlab function MISSION SERVER QDRONE POSITION CONTROL/Extract Vehicle Data/Extract Object Data ==
  data: data input double; position output double; orientation output double; index input double; tracking output double
function [position, orientation, tracking] = fcn(data, index)

n = length(data)/7;

if (index<=0)||(index>n)
    position = zeros(1,3); orientation = zeros(1,3); tracking = 0;
else
    position = [data(index*3-2), data(index*3-1), data(index*3)];
    orientation = [data((index+n)*3 - 2), data((index+n)*3 - 1), data((index+n)*3)];
    tracking = data(index + (n*6));
end

== matlab function Communication/Detect Communication loss/MATLAB Function ==
  data: time input double; stream_connection_loss output double; state input double; error input double
function stream_connection_loss  = fcn(time, state, error)

stream_connection_loss = 0;
if time > 1
    if ~((state == 2)&&(error >= 0))
        % stream connection is not established correctly
        stream_connection_loss = 1;
    end
end
